simulink model "stepMotor"  (Simulink 6.1)
settings: Solver=ode45  StartTime=0.0  StopTime=10.0  RelTol=1e-3
settings Model: LastModifiedBy=okawa
settings DebuggingCC: SolverPrmCheckMsg=warning

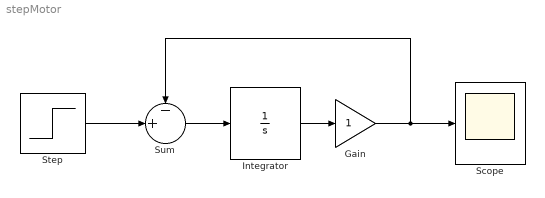
== system stepMotor ==
  Gain : Gain
  Integrator : Integrator
  Scope : Scope
  Step : Step  SampleTime=0
  Sum : Sum  Inputs=-+|
  wires:
  Sum/1 -> Integrator/1
  Integrator/1 -> Gain/1
  Step/1 -> Sum/2
  Gain/1 -> Sum/1, Scope/1
